simulink model "SimulationLQR_Linear"  (R2024b)
settings: Solver=VariableStepAuto  StartTime=0.0  StopTime=10  MaxStep=0.01  RelTol=1e-10
undefined symbols (not defined in the file): A, B, C, D, K
settings Model: Creator=Igor  LastModifiedBy=ybern

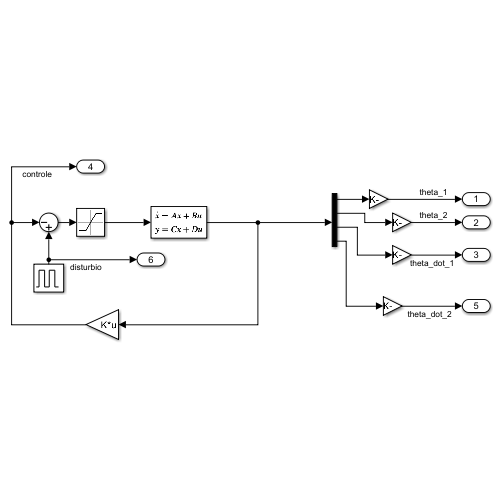
[thumbnail: Simulink's stored preview of the top-level diagram]
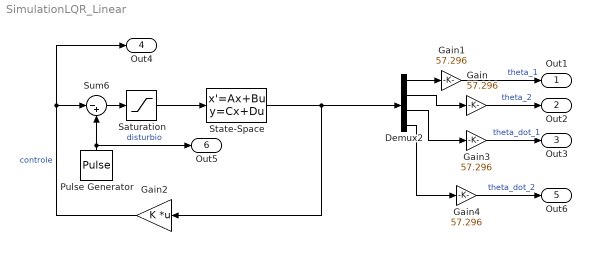
== system SimulationLQR_Linear ==
  Demux2 : Demux
  Gain{,1,3..4} (4 alike) : Gain  Gain=57.296
  Gain2 : Gain  Gain=K  Multiplication=Matrix(K*u)
  Pulse Generator : DiscretePulseGenerator  PulseType=Time based  Amplitude=0.5  PulseWidth=0.03  PhaseDelay=1
  Saturation : Saturate  UpperLimit=12  LowerLimit=-12
  State-Space : StateSpace  A=A  B=B  C=C  D=D  InitialCondition=[0, 0, 0, 0]
  Sum6 : Sum  Inputs=|-+
  Out1 : Outport
  Out2 : Outport  Port=2
  Out3 : Outport  Port=3
  Out4 : Outport  Port=4
  Out6 : Outport  Port=5
  Out5 : Outport  Port=6
  wires:
  Demux2/3 -> Gain3/1
  Sum6/1 -> Saturation/1
  Gain2/1 -> Sum6/1, Out4/1  "controle"
  Demux2/1 -> Gain1/1
  Demux2/2 -> Gain/1
  Gain/1 -> Out2/1  "theta_2"
  Gain1/1 -> Out1/1  "theta_1"
  Demux2/4 -> Gain4/1
  Gain3/1 -> Out3/1  "theta_dot_1"
  Gain4/1 -> Out6/1  "theta_dot_2"
  State-Space/1 -> Gain2/1, Demux2/1
  Pulse Generator/1 -> Out5/1, Sum6/2  "disturbio"
  Saturation/1 -> State-Space/1
